simulink model "mariner_sim"  (R2018b)
(part 6 of 22)

      mask Display: e = 0.06;c1 = [120 150 230]/255;c2 = ([120 150 230]+0)/383;c3 = ([120 150 230]+128)/383;patch([0 1 1 0],[0 0 1 1],c1);patch([0 1 1 1-e 1-e 0+e],[0 0 1 1-e 0+e 0+e],c2);patch([0 0 1 1-e 0+e 0+e],[0 1 1 1-e 1-e 0+e],c3);plot([0 1 1 0 0],[0 0 1 1 0]);disp('weights');
  "IW{3,2}(7,:)'" : Constant  Value=[-0.07566904451007912257853860182876815088093280792236328125;0.1764664757297027819493706601861049421131610870361328125;-0.364499912250532964730354024140979163348674774169921875;0.25215075287098642764505029845167882740497589111328125;-0.1000060372618759296781121292951866053044795989990234375;0.381923830188442614552712939257617108523845672607421875;-0.045850299756741506873591873727491474710404872894287109375;0.047864796286055423524263829904157319106161594390869140625;-0.06643349636241833999772410379591747187077999114990234375;0.1634532815131025385024798879385343752801418304443359375;0.346640369139526283159824515678337775170803070068359375;-0.08680651512990344986775426150416024029254913330078125;0.419712489527000409683665793636464513838291168212890625;-0.0377469643322714543121065844388795085251331329345703125;0.31890024231550173627880440108128823339939117431640625;0.1894278948513632709893528272004914470016956329345703125;-0.2293371712964074882190601556430920027196407318115234375;0.044325618369197607171461328334771678782999515533447265625;-0.0871809705177178095869550134011660702526569366455078125;-0.09963256325955148484663226327029406093060970306396484375;0.10084294619502286172174621015074080787599086761474609375;-0.08127514728793451548316539856386953033506870269775390625;-0.1708463567412454586769143816127325408160686492919921875;-0.221596252269772142629022937398985959589481353759765625;0.0521214250468912398961407461683847941458225250244140625;0.196020442729324451125449968458269722759723663330078125;-0.0908730578946762290737382272709510289132595062255859375;-0.27154741058105258399990589168737642467021942138671875;-0.2576922971409418838817373398342169821262359619140625;-0.396148828069049552258462654208415187895298004150390625;0.312905811193882055221138216438703238964080810546875;-0.2224454434672572256115330446846201084554195404052734375;-0.061862769650891498429690074090103735215961933135986328125;-0.31403917113093104962473489649710245430469512939453125;-0.2935458788371991811771977154421620070934295654296875;-0.0265161266431593566073043888309257454238831996917724609375;0.058519408039808061550157702868091291747987270355224609375;0.280596880864012521161754420973011292517185211181640625;-0.29776922773444847170054572416120208799839019775390625;0.2055720870071167938331058167023002170026302337646484375;-0.384794731920343358044789283667341805994510650634765625;-0.454912761402648413433524865467916242778301239013671875;-0.170435213621052350507767414455884136259555816650390625;-0.06595336538483138888455670212351833470165729522705078125;0.04172213390288710688214024457920459099113941192626953125;0.331879117390144806609697525345836766064167022705078125;-0.039307340499866748328994248140588751994073390960693359375;0.35648912085860384735269690281711518764495849609375]
      mask Display: e = 0.06;c1 = [120 150 230]/255;c2 = ([120 150 230]+0)/383;c3 = ([120 150 230]+128)/383;patch([0 1 1 0],[0 0 1 1],c1);patch([0 1 1 1-e 1-e 0+e],[0 0 1 1-e 0+e 0+e],c2);patch([0 0 1 1-e 0+e 0+e],[0 1 1 1-e 1-e 0+e],c3);plot([0 1 1 0 0],[0 0 1 1 0]);disp('weights');
  "IW{3,2}(8,:)'" : Constant  Value=[0.260855267964043402439955343652400188148021697998046875;0.1959474788465409289539564952065120451152324676513671875;-0.18939027337945113504957816985552199184894561767578125;-0.2058016744487644877903420592701877467334270477294921875;-0.09535149457185264354475151549195288680493831634521484375;-0.1546846155064123262690145566011779010295867919921875;-0.216200769491934396970833631712594069540500640869140625;0.11531785407635909701529186577317886985838413238525390625;-0.3391844957851619657418495989986695349216461181640625;-0.07548250051270884164456020926081691868603229522705078125;0.314305758044018557217924580982071347534656524658203125;-0.07067861042076116484533798711709096096456050872802734375;0.26104154430206782944168253379757516086101531982421875;-0.336950711730259755416483358203549869358539581298828125;0.130282465186766727160971868215710856020450592041015625;-0.122997557966610993052114508827798999845981597900390625;-0.09571032839985461893039797587334760464727878570556640625;-0.1442734995196451597276876555042690597474575042724609375;0.0168471195746746175980756987655695411376655101776123046875;0.37119451163318473163599264807999134063720703125;-0.00979740887552436011398437898378688259981572628021240234375;-0.03942835429676698477674534615289303474128246307373046875;0.10508029468090805680358101881211041472852230072021484375;-0.1467891993235539427331559636513702571392059326171875;0.34833586727569121332948043345822952687740325927734375;-0.08520200468869452981035550465094274841248989105224609375;0.31458996467059885393524609753512777388095855712890625;0.2481803462690128636580766396946273744106292724609375;0.0878492889610831551028269359449041076004505157470703125;0.3489831737886925910885338453226722776889801025390625;0.10378754922669364280096715447143651545047760009765625;-0.1813605497869798244270356235574581660330295562744140625;0.36564773304959796718094366951845586299896240234375;0.0034959883170754403429458800900420101243071258068084716796875;-0.2896525931359146266430570904049091041088104248046875;0.366924512580216577450897830203757621347904205322265625;0.37771954841357879839591760173789225518703460693359375;0.09062367165755258469062027870677411556243896484375;0.29111795110117355545042983067105524241924285888671875;-0.1480564581772230992040562114198110066354274749755859375;0.0982524719830027148947948489876580424606800079345703125;0.320288544421756082858365743959438987076282501220703125;0.13502547532971875821061757960706017911434173583984375;-0.2107682123158811371421705871398444287478923797607421875;-0.040758671728240984666324919771795975975692272186279296875;-0.1563092884851429442694126237256568856537342071533203125;-0.36046513100060695311555036823847331106662750244140625;-0.016084519152748451287227027250992250628769397735595703125]
      mask Display: e = 0.06;c1 = [120 150 230]/255;c2 = ([120 150 230]+0)/383;c3 = ([120 150 230]+128)/383;patch([0 1 1 0],[0 0 1 1],c1);patch([0 1 1 1-e 1-e 0+e],[0 0 1 1-e 0+e 0+e],c2);patch([0 0 1 1-e 0+e 0+e],[0 1 1 1-e 1-e 0+e],c3);plot([0 1 1 0 0],[0 0 1 1 0]);disp('weights');
  "IW{3,2}(9,:)'" : Constant  Value=[-0.0355083777042328463391385184877435676753520965576171875;-0.1083469422343521226803630952417734079062938690185546875;0.0131803557597451014016254333682809374295175075531005859375;-0.154123962529469249460589708178304135799407958984375;-0.06501369656356924264795082990531227551400661468505859375;-0.327213724984353249158886001168866641819477081298828125;0.052022389557672611692940023431219742633402347564697265625;-0.152590979299245088629533029234153218567371368408203125;0.257026431332516624994610765497782267630100250244140625;-0.05656358999492504258110869841402745805680751800537109375;0.257402745832333634812272293856949545443058013916015625;0.070696842089276235032713202599552460014820098876953125;-0.1968048088331234846126704951529973186552524566650390625;0.39541718419546934004671356888138689100742340087890625;0.11671659923560438743006528738987981341779232025146484375;-0.401356191998039346646720559874665923416614532470703125;-0.052044564827018614805442808801672072149813175201416015625;-0.437176290387372434853574532098718918859958648681640625;0.1028630840285027214786595095574739389121532440185546875;-0.395386835183042906205486133330850861966609954833984375;0.405653762310400678448019107236177660524845123291015625;0.37928354366156058485870516960858367383480072021484375;0.08700203387652395703444341279464424587786197662353515625;-0.201712967832759770825390432946733199059963226318359375;-0.302220739892191947451038913641241379082202911376953125;-0.1261720007615425576119605466374196112155914306640625;-0.022027808934258714945730872614149120636284351348876953125;-0.08199882881136082157791378222100320272147655487060546875;-0.16225635733624954593068423491786234080791473388671875;0.084559226794634401169759030381101183593273162841796875;-0.12350506422164285458276111739905900321900844573974609375;-0.01304867524767645663164028491110002505593001842498779296875;0.187438874454252724088831882909289561212062835693359375;-0.25370688800048857292068760216352529823780059814453125;0.4207600088669778415351174771785736083984375;0.0440277758757950665735592110650031827390193939208984375;0.07976282169325420168259910269625834189355373382568359375;-0.1294109975831389813816230116572114638984203338623046875;-0.1724065885765924954764471976886852644383907318115234375;-0.1970758444315297841509249110458767972886562347412109375;-0.2509718538410077304234846451436169445514678955078125;0.314320623315223424132369700600975193083286285400390625;0.2337879704639133915389237472481909207999706268310546875;0.265520190868665573180606997993891127407550811767578125;-0.102291244611242670980999491803231649100780487060546875;0.369965848733489754973646768121398054063320159912109375;-0.153636667995069420289411254998412914574146270751953125;-0.2081024945581331220267884418717585504055023193359375]
      mask Display: e = 0.06;c1 = [120 150 230]/255;c2 = ([120 150 230]+0)/383;c3 = ([120 150 230]+128)/383;patch([0 1 1 0],[0 0 1 1],c1);patch([0 1 1 1-e 1-e 0+e],[0 0 1 1-e 0+e 0+e],c2);patch([0 0 1 1-e 0+e 0+e],[0 1 1 1-e 1-e 0+e],c3);plot([0 1 1 0 0],[0 0 1 1 0]);disp('weights');
  Mux : Mux  Inputs=48
      mask Display: e = 0.06;c1 = [120 150 230]/255;c2 = ([120 150 230]+0)/383;c3 = ([120 150 230]+128)/383;patch([0 1 1 0],[0 0 1 1],c1);patch([0 1 1 1-e 1-e 0+e],[0 0 1 1-e 0+e 0+e],c2);patch([0 0 1 1-e 0+e 0+e],[0 1 1 1-e 1-e 0+e],c3);plot([0 1 1 0 0],[0 0 1 1 0]);disp('Mux');
  dotprod{1..48} (48 alike) : neural/Weight Functions/dotprod
  "lz{3,2}" : Outport
      mask Display: e = 0.06;c1 = [120 230 180]/255;c2 = ([120 230 180]+0)/(256+128);c3 = ([120 230 180]+128)/(256+128);patch([0 1 1 0],[0 0 1 1],c1);patch([0 1 1 1-e 1-e 0+e],[0 0 1 1-e 0+e 0+e],c2);patch([0 0 1 1-e 0+e 0+e],[0 1 1 1-e 1-e 0+e],c3);plot([0 1 1 0 0],[0 0 1 1 0]);
  wires:
  Mux/1 -> "lz{3,2}"/1
  dotprod48/1 -> Mux/48
  "IW{3,2}(48,:)'"/1 -> dotprod48/1
  dotprod47/1 -> Mux/47
  "IW{3,2}(47,:)'"/1 -> dotprod47/1
  dotprod46/1 -> Mux/46
  "IW{3,2}(46,:)'"/1 -> dotprod46/1
  dotprod45/1 -> Mux/45
  "IW{3,2}(45,:)'"/1 -> dotprod45/1
  dotprod44/1 -> Mux/44
  "IW{3,2}(44,:)'"/1 -> dotprod44/1
  dotprod43/1 -> Mux/43
  "IW{3,2}(43,:)'"/1 -> dotprod43/1
  dotprod42/1 -> Mux/42
  "IW{3,2}(42,:)'"/1 -> dotprod42/1
  dotprod41/1 -> Mux/41
  "IW{3,2}(41,:)'"/1 -> dotprod41/1
  dotprod40/1 -> Mux/40
  "IW{3,2}(40,:)'"/1 -> dotprod40/1
  dotprod39/1 -> Mux/39
  "IW{3,2}(39,:)'"/1 -> dotprod39/1
  dotprod38/1 -> Mux/38
  "IW{3,2}(38,:)'"/1 -> dotprod38/1
  dotprod37/1 -> Mux/37
  "IW{3,2}(37,:)'"/1 -> dotprod37/1
  dotprod36/1 -> Mux/36
  "IW{3,2}(36,:)'"/1 -> dotprod36/1
  dotprod35/1 -> Mux/35
  "IW{3,2}(35,:)'"/1 -> dotprod35/1
  dotprod34/1 -> Mux/34
  "IW{3,2}(34,:)'"/1 -> dotprod34/1
  dotprod33/1 -> Mux/33
  "IW{3,2}(33,:)'"/1 -> dotprod33/1
  dotprod32/1 -> Mux/32
  "IW{3,2}(32,:)'"/1 -> dotprod32/1
  dotprod31/1 -> Mux/31
  "IW{3,2}(31,:)'"/1 -> dotprod31/1
  dotprod30/1 -> Mux/30
  "IW{3,2}(30,:)'"/1 -> dotprod30/1
  dotprod29/1 -> Mux/29
  "IW{3,2}(29,:)'"/1 -> dotprod29/1
  dotprod28/1 -> Mux/28
  "IW{3,2}(28,:)'"/1 -> dotprod28/1
  dotprod27/1 -> Mux/27
  "IW{3,2}(27,:)'"/1 -> dotprod27/1
  dotprod26/1 -> Mux/26
  "IW{3,2}(26,:)'"/1 -> dotprod26/1
  dotprod25/1 -> Mux/25
  "IW{3,2}(25,:)'"/1 -> dotprod25/1
  dotprod24/1 -> Mux/24
  "IW{3,2}(24,:)'"/1 -> dotprod24/1
  dotprod23/1 -> Mux/23
  "IW{3,2}(23,:)'"/1 -> dotprod23/1
  dotprod22/1 -> Mux/22
  "IW{3,2}(22,:)'"/1 -> dotprod22/1
  dotprod21/1 -> Mux/21
  "IW{3,2}(21,:)'"/1 -> dotprod21/1
  dotprod20/1 -> Mux/20
  "IW{3,2}(20,:)'"/1 -> dotprod20/1
  dotprod19/1 -> Mux/19
  "IW{3,2}(19,:)'"/1 -> dotprod19/1
  dotprod18/1 -> Mux/18
  "IW{3,2}(18,:)'"/1 -> dotprod18/1
  dotprod17/1 -> Mux/17
  "IW{3,2}(17,:)'"/1 -> dotprod17/1
  dotprod16/1 -> Mux/16
  "IW{3,2}(16,:)'"/1 -> dotprod16/1
  dotprod15/1 -> Mux/15
  "IW{3,2}(15,:)'"/1 -> dotprod15/1
  dotprod14/1 -> Mux/14
  "IW{3,2}(14,:)'"/1 -> dotprod14/1
  dotprod13/1 -> Mux/13
  "IW{3,2}(13,:)'"/1 -> dotprod13/1
  dotprod12/1 -> Mux/12
  "IW{3,2}(12,:)'"/1 -> dotprod12/1
  dotprod11/1 -> Mux/11
  "IW{3,2}(11,:)'"/1 -> dotprod11/1
  dotprod10/1 -> Mux/10
  "IW{3,2}(10,:)'"/1 -> dotprod10/1
  dotprod9/1 -> Mux/9
  "IW{3,2}(9,:)'"/1 -> dotprod9/1
  dotprod8/1 -> Mux/8
  "IW{3,2}(8,:)'"/1 -> dotprod8/1
  dotprod7/1 -> Mux/7
  "IW{3,2}(7,:)'"/1 -> dotprod7/1
  dotprod6/1 -> Mux/6
  "IW{3,2}(6,:)'"/1 -> dotprod6/1
  dotprod5/1 -> Mux/5
  "IW{3,2}(5,:)'"/1 -> dotprod5/1
  dotprod4/1 -> Mux/4
  "IW{3,2}(4,:)'"/1 -> dotprod4/1
  dotprod3/1 -> Mux/3
  "IW{3,2}(3,:)'"/1 -> dotprod3/1
  dotprod2/1 -> Mux/2
  "IW{3,2}(2,:)'"/1 -> dotprod2/1
  dotprod1/1 -> Mux/1
  "ad{3,2}"/1 -> dotprod48/2, dotprod47/2, dotprod46/2, dotprod45/2, dotprod44/2, dotprod43/2, dotprod42/2, dotprod41/2, dotprod40/2, dotprod39/2, dotprod38/2, dotprod37/2, dotprod36/2, dotprod35/2, dotprod34/2, dotprod33/2, dotprod32/2, dotprod31/2, dotprod30/2, dotprod29/2, dotprod28/2, dotprod27/2, dotprod26/2, dotprod25/2, dotprod24/2, dotprod23/2, dotprod22/2, dotprod21/2, dotprod20/2, dotprod19/2, dotprod18/2, dotprod17/2, dotprod16/2, dotprod15/2, dotprod14/2, dotprod13/2, dotprod12/2, dotprod11/2, dotprod10/2, dotprod9/2, dotprod8/2, dotprod7/2, dotprod6/2, dotprod5/2, dotprod4/2, dotprod3/2, dotprod2/2, dotprod1/2
  "IW{3,2}(1,:)'"/1 -> dotprod1/1
